simulink model "test"  (Simulink 8.4)
settings: Solver=ode45  StartTime=0.0  StopTime=1  RelTol=1e-3
undefined symbols (not defined in the file): a, Gn, Ipvn, Iscn, k, Ki, Kv, Npp, Ns, Nss, q, Rp, Rs, Tn, Vocn
libraries: powerlib x14, simulink x1
settings Model: Creator=SELVA  LastModifiedBy=SELVA

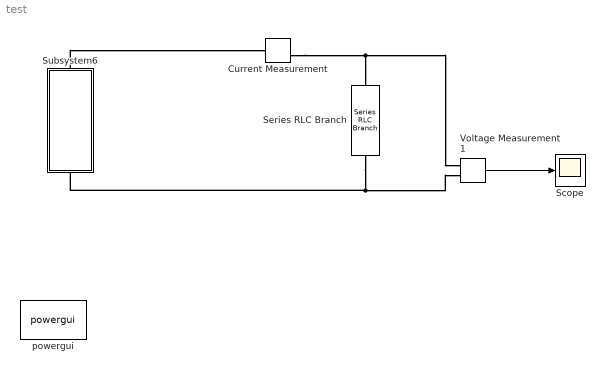
== system test ==
  Current Measurement : powerlib/Measurements/Current Measurement  PhasorSimulation=off  OutputType=Complex  PSBequivalent=0
  Scope : Scope
  Series RLC Branch : powerlib/Elements/Series RLC Branch  LConnTagsString=__new0  RConnTagsString=__new0  BranchType=R  Resistance=100  Inductance=1e-3  SetiL0=off  InitialCurrent=0  Capacitance=1e-6  Setx0=off  InitialVoltage=0  Measurements=None
  Subsystem6 : Subsystem
  Voltage Measurement1 : powerlib/Measurements/Voltage Measurement  PhasorSimulation=off  OutputType=Complex  PSBequivalent=0
  powergui : powerlib/powergui  Priority=1  SimulationMode=Discrete  SolverType=Tustin/Backward Euler (TBE)  SampleTime=5e-5  frequency=60  SPID=off  DisableSnubberDevices=off  DisableRonSwitches=off  DisableVfSwitches=off  SwTol=0  DisplayEquations=off  Interpol=off  methode=off  Ts=0  frequencyindice=0  Pbase=100e6  ErrMax=1e-4  Iterations=50  UnitsV=kV  UnitsW=MW  FunctionMessages=off  echomessages=off  HookPort=off  EnableUseOfTLC=off  x0status=blocks  RestoreLinks=warning  ResistiveCurrentMeasurement=off  Frange=[0:2:500]  Ylog=off  Xlog=on  ShowGrid=off  save=off  variable=ZData  structure=0  ZoomFFT=off  StartTime=0.0  cycles=1  DisplayStyle=1  fundamental=60  FreqAxis=off  MaxFrequency=1000  frequencyindicesteady=1  RmsSteady=1  display=off
  wires:
  Voltage Measurement1/1 -> Scope/1
  connections:
  Series RLC Branch/RConn1 -- Subsystem6/RConn1 -- Voltage Measurement1/LConn2
  Subsystem6/LConn1 -- Current Measurement/LConn1
  Current Measurement/RConn1 -- Series RLC Branch/LConn1 -- Voltage Measurement1/LConn1

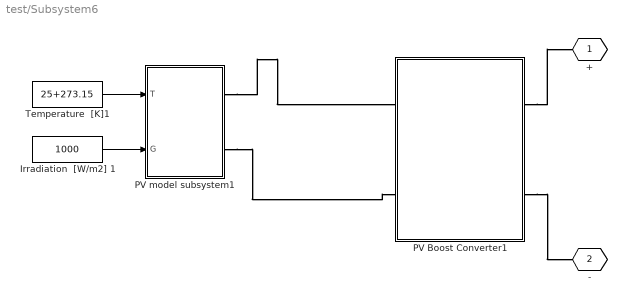
== system test/Subsystem6 ==
  Irradiation  [W/m2] 1 : Constant  Value=1000
  PV Boost Converter1 : Subsystem
  PV model subsystem1 : Subsystem
  Temperature  [K]1 : Constant  Value=25+273.15
  + : PMIOPort  Port=1  Side=Left
  - : PMIOPort  Port=2  Side=Right
  wires:
  Temperature  [K]1/1 -> PV model subsystem1/1(T)
  Irradiation  [W/m2] 1/1 -> PV model subsystem1/2(G)
  connections:
  PV Boost Converter1/RConn1 -- +/RConn1
  PV Boost Converter1/RConn2 -- -/RConn1
  PV model subsystem1/RConn2 -- PV Boost Converter1/LConn2
  PV model subsystem1/RConn1 -- PV Boost Converter1/LConn1

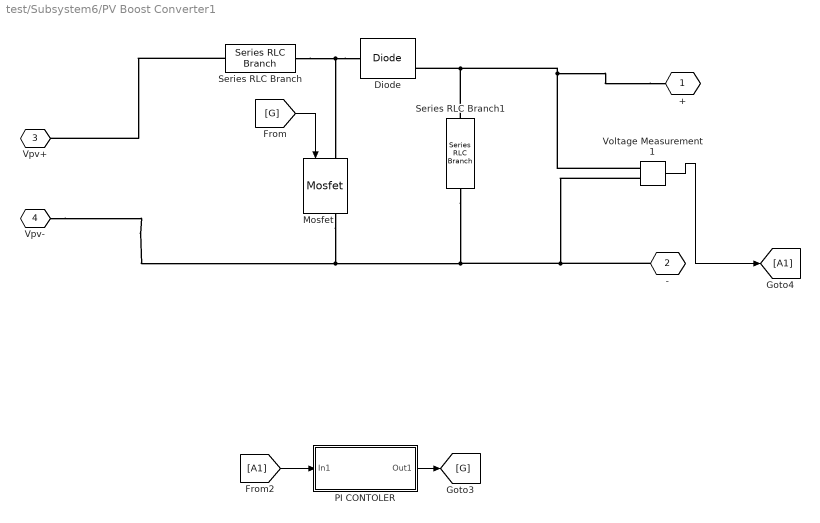
== system test/Subsystem6/PV Boost Converter1 ==
  Diode : powerlib/Power Electronics/Diode  Ron=0.001  Lon=0  Vf=0.8  IC=0  UseSnubber=off  Rs=500  Cs=250e-9  Measurements=on
  Mosfet : powerlib/Power Electronics/Mosfet  Ron=0.1  Lon=0  Rd=0.01  Vfd=0  IC=0  Rs=1e5  Cs=inf  Measurements=on
  PI CONTOLER : Subsystem
  Series RLC Branch : powerlib/Elements/Series RLC Branch  LConnTagsString=__new0  RConnTagsString=__new0  BranchType=L  Resistance=1  Inductance=1e-3  SetiL0=off  InitialCurrent=0  Capacitance=1e-6  Setx0=off  InitialVoltage=0  Measurements=None
  Series RLC Branch1 : powerlib/Elements/Series RLC Branch  LConnTagsString=__new0  RConnTagsString=__new0  BranchType=C  Resistance=1  Inductance=12e-3  SetiL0=off  InitialCurrent=0  Capacitance=1000e-6  Setx0=off  InitialVoltage=0  Measurements=None
  Voltage Measurement1 : powerlib/Measurements/Voltage Measurement  PhasorSimulation=off  OutputType=Complex  PSBequivalent=0
  + : PMIOPort  Port=1  Side=Right
  - : PMIOPort  Port=2  Side=Right
  Vpv+ : PMIOPort  Tag=PMCPort  Port=3  Side=Left
  Vpv- : PMIOPort  Tag=PMCPort  Port=4  Side=Left
  wires:
  [A1] -> PI CONTOLER/1(In1)
  PI CONTOLER/1(Out1) -> [G]
  [G] -> Mosfet/1
  Voltage Measurement1/1 -> [A1]
  connections:
  +/RConn1 -- Diode/RConn1 -- Series RLC Branch1/LConn1 -- Voltage Measurement1/LConn1
  Vpv-/RConn1 -- -/RConn1 -- Voltage Measurement1/LConn2 -- Series RLC Branch1/RConn1 -- Mosfet/RConn1
  Diode/LConn1 -- Mosfet/LConn1 -- Series RLC Branch/RConn1
  Series RLC Branch/LConn1 -- Vpv+/RConn1

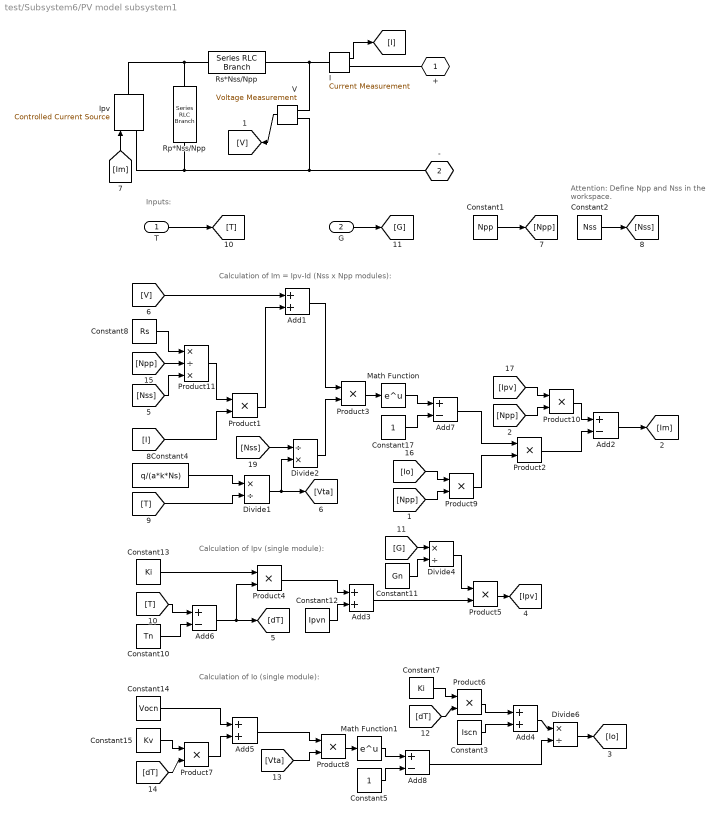
== system test/Subsystem6/PV model subsystem1 ==
  note: Inputs:
  note: Calculation of Im = Ipv-Id (Nss x Npp modules):
  note: Calculation of Ipv (single module):
  note: Calculation of Io (single module):
  note: Attention:
      |
      | Define Npp and Nss in the workspace.
  T : Inport
  G : Inport  Port=2
  Add{1,3..5} (4 alike) : Sum
  Add{2,6..8} (4 alike) : Sum  Inputs=+-
  Constant1 : Constant  Value=Npp
  Constant10 : Constant  Value=Tn
  Constant11 : Constant  Value=Gn
  Constant12 : Constant  Value=Ipvn
  Constant13 : Constant  Value=Ki
  Constant14 : Constant  Value=Vocn
  Constant15 : Constant  Value=Kv
  Constant17 : Constant
  Constant2 : Constant  Value=Nss
  Constant3 : Constant  Value=Iscn
  Constant4 : Constant  Value=q/(a*k*Ns)
  Constant5 : Constant
  Constant7 : Constant  Value=Ki
  Constant8 : Constant  Value=Rs
  Divide1 : Product  Inputs=*/
  Divide2 : Product  Inputs=/*
  Divide4 : Product  Inputs=*/
  Divide6 : Product  Inputs=*/
  I : powerlib/Measurements/Current Measurement  PhasorSimulation=off  OutputType=Complex  PSBequivalent=0
  Ipv : powerlib/Electrical Sources/Controlled Current Source  Initialize=on  Source_Type=DC  Amplitude=0  Phase=0  Frequency=0  Measurements=None
  Math Function : Math  SaturateOnIntegerOverflow=on
  Math Function1 : Math  SaturateOnIntegerOverflow=on
  Product{1..10} (10 alike) : Product  RndMeth=Zero
  Product11 : Product  Inputs=*/*  RndMeth=Zero
  Rp*Nss/Npp : powerlib/Elements/Series RLC Branch  LConnTagsString=__new0  RConnTagsString=__new0  BranchType=R  Resistance=Rp*Nss/Npp  Inductance=1e-3  SetiL0=off  InitialCurrent=0  Capacitance=1e-6  Setx0=off  InitialVoltage=0  Measurements=None
  Rs*Nss/Npp : powerlib/Elements/Series RLC Branch  LConnTagsString=__new0  RConnTagsString=__new0  BranchType=R  Resistance=Rs*Nss/Npp  Inductance=1e-3  SetiL0=off  InitialCurrent=0  Capacitance=1e-6  Setx0=off  InitialVoltage=0  Measurements=None
  "V " : powerlib/Measurements/Voltage Measurement  PhasorSimulation=off  OutputType=Complex  PSBequivalent=0
  + : PMIOPort  Port=1  Side=Right
  - : PMIOPort  Port=2  Side=Right
  wires:
  I/1 -> [I]
  "V "/1 -> [V]
  [Im] -> Ipv/1
  G/1 -> [G]
  T/1 -> [T]
  Constant10/1 -> Add6/2
  [T] -> Add6/1
  [I] -> Product1/2
  Constant4/1 -> Divide1/1
  [T] -> Divide1/2
  [V] -> Add1/1
  Product3/1 -> Math Function/1
  Add2/1 -> [Im]
  Add1/1 -> Product3/1
  [G] -> Divide4/1
  Constant11/1 -> Divide4/2
  Constant13/1 -> Product4/1
  [dT] -> Product6/2
  Constant7/1 -> Product6/1
  [dT] -> Product7/2
  Constant14/1 -> Add5/1
  Product8/1 -> Math Function1/1
  Add5/1 -> Product8/1
  Constant17/1 -> Add7/2
  Add7/1 -> Product2/1
  Constant5/1 -> Add8/2
  Math Function1/1 -> Add8/1
  Divide6/1 -> [Io]
  Product5/1 -> [Ipv]
  Product1/1 -> Add1/2
  Math Function/1 -> Add7/1
  Product4/1 -> Add3/1
  Add3/1 -> Product5/2
  Divide4/1 -> Product5/1
  Product7/1 -> Add5/2
  Constant15/1 -> Product7/1
  [Vta] -> Product8/2
  Add8/1 -> Divide6/2
  Constant3/1 -> Add4/2
  Product6/1 -> Add4/1
  Constant12/1 -> Add3/2
  Product2/1 -> Add2/2
  Product9/1 -> Product2/2
  [Io] -> Product9/1
  [Npp] -> Product9/2
  Constant1/1 -> [Npp]
  Constant2/1 -> [Nss]
  [Ipv] -> Product10/1
  [Npp] -> Product10/2
  Product10/1 -> Add2/1
  Constant8/1 -> Product11/1
  [Npp] -> Product11/2
  [Nss] -> Product11/3
  Product11/1 -> Product1/1
  [Nss] -> Divide2/1
  Divide1/1 -> Divide2/2, [Vta]
  Divide2/1 -> Product3/2
  Add6/1 -> [dT], Product4/2
  Add4/1 -> Divide6/1
  connections:
  I/LConn1 -- "V "/LConn1 -- Rs*Nss/Npp/RConn1
  -/RConn1 -- Rp*Nss/Npp/RConn1 -- Ipv/LConn1 -- "V "/LConn2
  Ipv/RConn1 -- Rs*Nss/Npp/LConn1 -- Rp*Nss/Npp/LConn1
  +/RConn1 -- I/RConn1

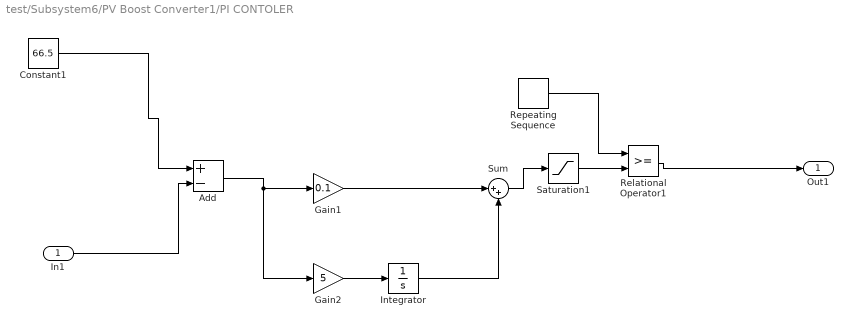
== system test/Subsystem6/PV Boost Converter1/PI CONTOLER ==
  In1 : Inport
  Add : Sum  Inputs=+-
  Constant1 : Constant  Value=66.5
  Gain1 : Gain  Gain=0.1
  Gain2 : Gain  Gain=5
  Integrator : Integrator
  Relational Operator1 : RelationalOperator  OutDataTypeStr=boolean
  Repeating Sequence : simulink/Sources/Repeating Sequence  rep_seq_t=[0 0.0001 0.0002]  rep_seq_y=[0 10 0]
  Saturation1 : Saturate  UpperLimit=10  LowerLimit=0
  Sum : Sum  Inputs=|++
  Out1 : Outport
  wires:
  Saturation1/1 -> Relational Operator1/2
  Gain2/1 -> Integrator/1
  Sum/1 -> Saturation1/1
  Integrator/1 -> Sum/2
  Gain1/1 -> Sum/1
  Relational Operator1/1 -> Out1/1
  Repeating Sequence/1 -> Relational Operator1/1
  Add/1 -> Gain2/1, Gain1/1
  Constant1/1 -> Add/1
  In1/1 -> Add/2
